simulink model "test"  (R2022b)
settings: Solver=VariableStepAuto  StartTime=0.0  StopTime=20  RelTol=1e-3
settings Model: Creator=yujiang  LastModifiedBy=yujiang
settings DataIOCC: ReturnWorkspaceOutputs=off

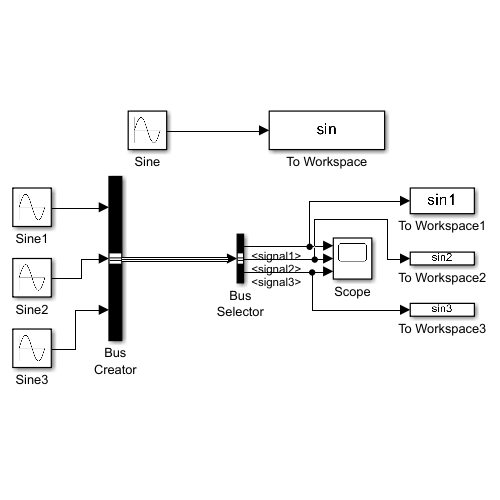
[thumbnail: Simulink's stored preview of the top-level diagram]
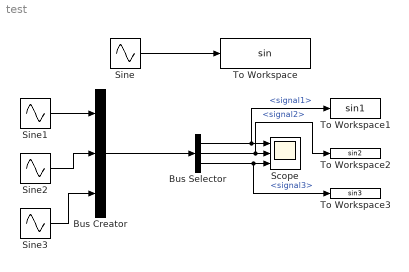
== system test ==
  Bus Creator : BusCreator  Inputs=3
  Bus Selector : BusSelector  OutputSignals=signal1,signal2,signal3
  Scope : Scope  NumInputPorts=3
  Sine : Sin  Amplitude=10  SampleTime=0
  Sine1 : Sin  Amplitude=10  SampleTime=0
  Sine2 : Sin  Amplitude=20  SampleTime=0
  Sine3 : Sin  Amplitude=30  SampleTime=0
  To Workspace : ToWorkspace  VariableName=sin  SampleTime=-1
  To Workspace1 : ToWorkspace  VariableName=sin1  SampleTime=-1
  To Workspace2 : ToWorkspace  VariableName=sin2  SampleTime=-1
  To Workspace3 : ToWorkspace  VariableName=sin3  SampleTime=-1
  wires:
  Sine/1 -> To Workspace/1
  Bus Creator/1 -> Bus Selector/1
  Sine1/1 -> Bus Creator/1
  Sine2/1 -> Bus Creator/2
  Sine3/1 -> Bus Creator/3
  Bus Selector/1 -> To Workspace1/1, Scope/1  "<signal1>"
  Bus Selector/2 -> To Workspace2/1, Scope/2  "<signal2>"
  Bus Selector/3 -> To Workspace3/1, Scope/3  "<signal3>"
